simulink model "prestoAJ_a448_Reentry_Sim"  (R2024b)
settings: Solver=VariableStepAuto  StartTime=0.0  StopTime=tspan  RelTol=1e-9
values from neighbouring files (symbols this model uses):
  Cd = 0.02723    [prestoAJ_a448_Reentry.m]
  CL = 0.11059    [prestoAJ_a448_Reentry.m]
  H = 7100    [prestoAJ_a448_Reentry.m]
  m_reentry = m_dry + m_prop*.05    (= 90200)    [prestoAJ_a448_Reentry.m]
  mu = 3.986004418e14    (= 398600441800000)    [prestoAJ_a448_Reentry.m]
  OmegaE = 7.2921159e-5    (= 7.2921159e-05)    [prestoAJ_a448_Reentry.m]
  rE = 6378000    [prestoAJ_a448_Reentry.m]
  rho0 = 1.225    [prestoAJ_a448_Reentry.m]
  S = 138    [prestoAJ_a448_Reentry.m]
  x0 = 0    [main_simulation.m]    (also in prestoAJ_a448_Reentry.m = [r0;lon0;lat0;v0;y0;psi0])
undefined symbols (not defined in the file or in its folder): r_ECI_0, v_ECI_0
libraries: simulink x1
settings Model: Creator=prest  LastModifiedBy=prest

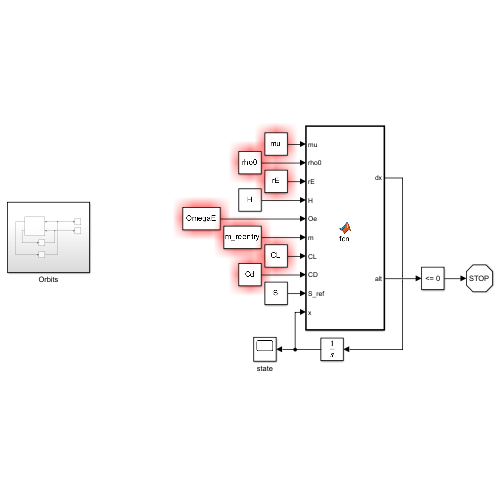
[thumbnail: Simulink's stored preview of the top-level diagram]
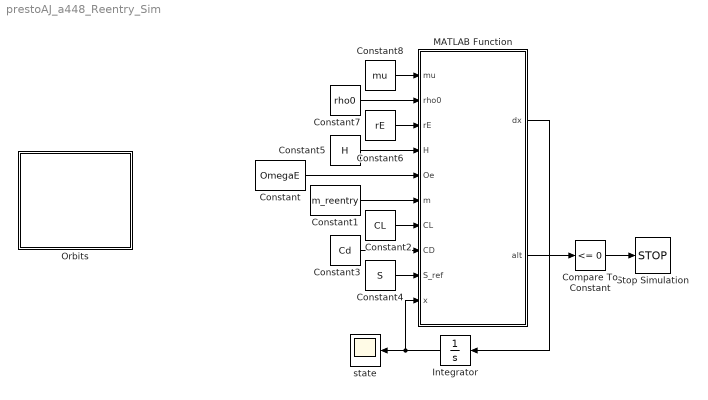
== system prestoAJ_a448_Reentry_Sim ==
  Compare To Constant : simulink/Logic and Bit Operations/Compare To Constant  relop=<=  const=0  OutDataTypeStr=boolean
  Constant : Constant  Value=OmegaE
  Constant1 : Constant  Value=m_reentry
  Constant2 : Constant  Value=CL
  Constant3 : Constant  Value=Cd
  Constant4 : Constant  Value=S
  Constant5 : Constant  Value=H
  Constant6 : Constant  Value=rE
  Constant7 : Constant  Value=rho0
  Constant8 : Constant  Value=mu
  Integrator : Integrator  InitialCondition=x0
  MATLAB Function : MATLAB Function  TreatAsAtomicUnit=on
  Orbits : Subsystem
  Stop Simulation : Stop
  state : Scope
  wires:
  Integrator/1 -> MATLAB Function/10(x), state/1
  MATLAB Function/1(dx) -> Integrator/1
  Constant/1 -> MATLAB Function/5(Oe)
  Constant1/1 -> MATLAB Function/6(m)
  Constant2/1 -> MATLAB Function/7(CL)
  Constant3/1 -> MATLAB Function/8(CD)
  Constant4/1 -> MATLAB Function/9(S_ref)
  Constant5/1 -> MATLAB Function/4(H)
  Constant6/1 -> MATLAB Function/3(rE)
  Constant7/1 -> MATLAB Function/2(rho0)
  Constant8/1 -> MATLAB Function/1(mu)
  MATLAB Function/2(alt) -> Compare To Constant/1
  Compare To Constant/1 -> Stop Simulation/1

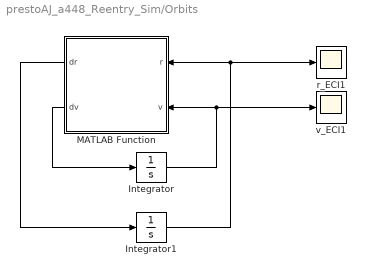
== system prestoAJ_a448_Reentry_Sim/Orbits ==
  Integrator : Integrator  InitialCondition=v_ECI_0
  Integrator1 : Integrator  InitialCondition=r_ECI_0
  MATLAB Function : MATLAB Function  TreatAsAtomicUnit=on
  r_ECI1 : Scope
  v_ECI1 : Scope
  wires:
  Integrator/1 -> v_ECI1/1, MATLAB Function/2(v)
  Integrator1/1 -> r_ECI1/1, MATLAB Function/1(r)
  MATLAB Function/1(dr) -> Integrator1/1
  MATLAB Function/2(dv) -> Integrator/1

== matlab function prestoAJ_a448_Reentry_Sim/MATLAB Function ==
  data: mu input; rho0 input; rE input; H input; Oe input; m input; CL input; CD input; S_ref input; dx output; x input; alt output
function [dx, alt]  = fcn(mu, rho0, rE, H, Oe, m, CL, CD, S_ref, x)

% Calculate/Declare Constants
sig = 0; % [rad] Bank angle (Might change location later)
rho = rho0*exp(-(x(1)-rE)/H); % [kg/m^3] Current Atmospheric Density
g = mu/(x(1))^2; % [m/s^2] Gravity at given altitude
L = 0.5*CL*rho*x(4)^2*S_ref;
D = 0.5*CD*rho*x(4)^2*S_ref;

% Calculate derivative of state vector
dx = zeros(6,1);
dx(1) = x(4)*sin(x(5));
dx(2) = x(4)*cos(x(5))*sin(x(6))/x(1)/cos(x(3));
dx(3) = x(4)*cos(x(5))*cos(x(6))/x(1);
dx(4) = -D/m - g*sin(x(5)) + Oe^2*x(1)*cos(x(3))*(sin(x(5))*cos(x(3))-cos(x(5))*sin(x(3))*cos(x(6)));
dx(5) = (L*cos(sig)/m - g*cos(x(5)) + x(4)^2*cos(x(5))/x(1) + 2*Oe*x(4)*cos(x(3))*sin(x(6)) + Oe^2*x(1)*cos(x(3))*(cos(x(5))*cos(x(3)) + sin(x(5))*cos(x(6))*sin(x(3))))/x(4);
dx(6) = (L*sin(sig)/m/cos(x(5)) + x(4)^2*cos(x(5))*sin(x(6))*tan(x(3))/x(1) -  2*Oe*x(4)*(tan(x(5))*cos(x(6))*cos(x(3)) - sin(x(3))) + Oe^2*x(1)*sin(x(6))*sin(x(3))*cos(x(3))/cos(x(5)))/x(4);

% Calculate altitude for termination conditition
alt = x(1)-rE;

== matlab function prestoAJ_a448_Reentry_Sim/Orbits/MATLAB Function ==
  data: r input; dr output; v input; dv output
function [dr,dv] = orbitalDynamics(r, v)
    mu = 398600;
    rnorm = norm(r);
    a = -mu.*r(:)./(rnorm^3);
    
    dr = v(:);
    dv = a(:);
